simulink library "visionanalysis"  (R2017b)
settings: Solver=ode45  StartTime=0.0  StopTime=10.0  RelTol=1e-3
undefined symbols (not defined in the file or in its folder): dtInfo, fspecial
libraries: visionstatistics x1
settings Model: FPTRunName=Active  ExtModeAutoUpdateStatusClock=off  Creator=The MathWorks, Inc.  LastModifiedBy=The MathWorks, Inc.
settings DataIOCC: LimitDataPoints=on  SaveFormat=Array  SignalLoggingSaveFormat=ModelDataLogs
settings OptimizationCC: BlockReduction=off  BooleanDataType=off  ExpressionDepthLimit=2147483647  EfficientMapNaN2IntZero=off  LifeSpan=inf
settings DebuggingCC: SaveWithParameterizedLinksMsg=none  UnderspecifiedInitializationDetection=Classic  MergeDetectMultiDrivingBlocksExec=none  SignalResolutionControl=TryResolveAllWithWarning  FcnCallInpInsideContextMsg=warning  AllowSymbolicDim=off  StateNameClashWarn=warning  StrictBusMsg=Warning  SFUnexpectedBacktrackingDiag=warning  SFNoUnconditionalDefaultTransitionDiag=warning  SFExecutionAtInitializationDiag=none
settings HardwareCC: ProdBitPerPointer=32  ProdBitPerSizeT=32  ProdBitPerPtrDiffT=32  ProdLargestAtomicFloat=None  ProdIntDivRoundTo=Undefined  ProdEndianess=Unspecified  ProdWordSize=32  ProdHWDeviceType=32-bit Generic  TargetUnknown=on
settings ModelReferenceCC: PropagateSignalLabelsOutOfModel=off
settings CodeAppCC: StateflowObjectComments=on
settings GRTTargetCC: TargetLangStandard=C89/C90 (ANSI)  GeneratePreprocessorConditionals=Disable all  CombineOutputUpdateFcns=off  GRTInterface=on
settings ConfigComp: CovMetricSettings=dw  CovHtmlReporting=on  CovSaveCumulativeToWorkspaceVar=on  CovSaveSingleToWorkspaceVar=on  CovShowResultsExplorer=off  CovExternalEMLEnable=off  CovSFcnEnable=off

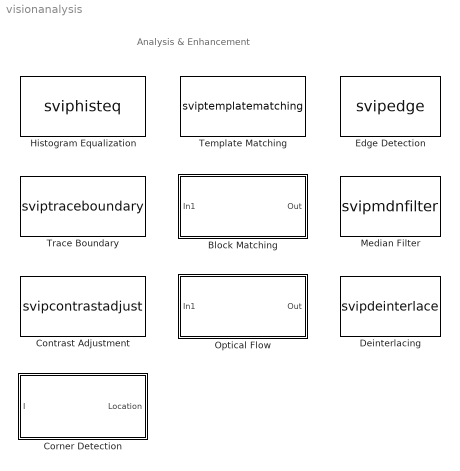
== system visionanalysis ==
  note: Analysis & Enhancement
  Block Matching : Subsystem  DialogController=vipDDGCreate  mask(Block Matching){which2img=Current frame and N-th frame back, N=1, searchMethod=Exhaustive, blockSize=[17 17], overlapping=[0 0], maxDisplacement=[7 7], matchCriteria=Mean square error (MSE), outVelForm=Magnitude-squared, outputMode=Binary point scaling, outputWordLength=8, outputFracLength=0, accumMode=Binary point scaling, accumWordLength=32, accumFracLength=0, prodOutputMode=Binary point scaling, prodOutputWordLength=32, prodOutputFracLength=0, roundingMode=Floor, overflowMode=on, LockScale=off}
      mask prompts: which2img "vision:masks:EstimateMotionBetween"; N "vision:masks:N"; searchMethod "vision:masks:SearchMethod"; blockSize "vision:masks:BlockSizeheightWidth"; overlapping "vision:masks:OverlapSizerC"; maxDisplacement "vision:masks:MaximumDisplacementrC"; matchCriteria "vision:masks:BlockMatchingCriteria"; outVelForm "vision:masks:VelocityOutput"; outputMode "vision:masks:FixedpointOutputAttributes"; outputWordLength "vision:masks:OutputWordLength"; outputFracLength "vision:masks:OutputFractionalLength"; accumMode "vision:masks:FixedpointAccumulatorAttributes"; accumWordLength "vision:masks:AccumulatorWordLength"; accumFracLength "vision:masks:AccumulatorFractionLength"; prodOutputMode "vision:masks:FixedpointProductOutputAttribute"; prodOutputWordLength "vision:masks:ProductOutputWordLength"; prodOutputFracLength "vision:masks:ProductOutputFractionLength"; roundingMode "vision:masks:RoundIntegerCalculationsTowards"; overflowMode "vision:masks:SaturateOnIntegerOverflow"; LockScale "vision:masks:LockScaling1"
      mask help: vision:masks:BlockMatchingDescription
      mask init:
      | [disp_str,si,so]=vipblkblockmatch('icon',which2img);
      | vipblkblockmatch('init');
      mask Help: eval('visionblockhelp');
      mask TypeOptions which2img: vision:masks:TwoImages | vision:masks:CurrentFrameAndNthFrameBack
      mask TypeOptions searchMethod: vision:masks:Exhaustive | vision:masks:Threestep
      mask TypeOptions matchCriteria: vision:masks:MeanSquareErrorMSE | vision:masks:MeanAbsoluteDifferenceMAD
      mask TypeOptions outVelForm: vision:masks:HorizontalAndVerticalComponentsI | vision:masks:Magnitudesquared
      mask TypeOptions outputMode: Binary point scaling | Slope and bias scaling
      mask TypeOptions accumMode: Binary point scaling | Slope and bias scaling
      mask TypeOptions prodOutputMode: Same as input | Binary point scaling | Slope and bias scaling
      mask TypeOptions roundingMode: dspshared:FixptDialog:Ceiling_CB | dspshared:FixptDialog:Convergent_CB | dspshared:FixptDialog:Floor_CB | dspshared:FixptDialog:Nearest_CB | dspshared:FixptDialog:Round_CB | dspshared:FixptDialog:Simplest_CB | dspshared:FixptDialog:Zero_CB
      mask Display:
      | disp(disp_str);
      | port_label('input',si(1).port,si(1).txt);
      | port_label('input',si(2).port,si(2).txt);
      | 
      | port_label('output',1,so(1).txt);
  Contrast Adjustment : S-Function  DialogController=vipDDGCreate  FunctionName=svipcontrastadjust  Parameters=methodInputRange, rangeIn, fracSaturate, isBinNum, binNum, methodOutputRange, rangeOut, prod1Mode, prod1WordLength, prod1FracLength, prod2Mode, prod2WordLength, prod2FracLength, dtInfo.roundingMode, dtInfo.overflowMode  SFunctionDeploymentMode=off  EnableBusSupport=off  mask(Contrast Adjustment){methodInputRange=Full input data range [min max], rangeIn=[0 255], fracSaturate=[1 1], isBinNum=on, binNum=256, methodOutputRange=Full data type range, rangeOut=[0 255], prod1Mode=Binary point scaling, prod1WordLength=32, prod1FracLength=16, prod2Mode=Binary point scaling, prod2WordLength=32, prod2FracLength=16, roundingMode=Floor, overflowMode=off, LockScale=off}
      mask prompts: methodInputRange "vision:masks:AdjustPixelValuesFrom"; rangeIn "vision:masks:RangelowHigh"; fracSaturate "vision:masks:PercentageOfPixelsToSaturatelowH"; isBinNum "vision:masks:SpecifyNumberOfHistogramBinsused"; binNum "vision:masks:NumberOfHistogramBins"; methodOutputRange "vision:masks:AdjustPixelValuesTo"; rangeOut "vision:masks:RangelowHigh"; prod1Mode "vision:masks:Product1Attributes"; prod1WordLength "vision:masks:Product1WordLength"; prod1FracLength "vision:masks:Product1FractionLength"; prod2Mode "vision:masks:Product2Attributes"; prod2WordLength "vision:masks:Product2WordLength"; prod2FracLength "vision:masks:Product2FractionLength"; roundingMode "vision:masks:RoundIntegerCalculationsToward"; overflowMode "vision:masks:SaturateOnIntegerOverflow"; LockScale "vision:masks:LockScaling1"
      mask help: vision:masks:ContrastAdjustmentDescription
      mask init:
      | dtInfo = dspGetFixptDataTypeInfo(gcbh,1);
      | fracSaturate = single(fracSaturate) ./ single(100);
      mask Help: eval('visionblockhelp');
      mask TypeOptions methodInputRange: vision:masks:FullInputDataRangeminMax | vision:masks:UserdefinedRange | vision:masks:RangeDeterminedBySaturating
      mask TypeOptions methodOutputRange: vision:masks:FullDataTypeRange | vision:masks:UserdefinedRange
      mask TypeOptions prod1Mode: Binary point scaling | Slope and bias scaling
      mask TypeOptions prod2Mode: Binary point scaling | Slope and bias scaling
      mask TypeOptions roundingMode: dspshared:FixptDialog:Ceiling_CB | dspshared:FixptDialog:Convergent_CB | dspshared:FixptDialog:Floor_CB | dspshared:FixptDialog:Nearest_CB | dspshared:FixptDialog:Round_CB | dspshared:FixptDialog:Simplest_CB | dspshared:FixptDialog:Zero_CB
      mask Display:
      | disp('Contrast\nAdjustment');
      | port_label('input',1,'I');
  Corner Detection : Subsystem  DialogController=vipDDGCreate  mask(Corner Detection){method=Harris corner detection (Harris & Stephens), factor=0.04, filter=fspecial('gaussian', [1 5], 1.5), thrInten=0.1, thrAngle=157.5, output=Obsolete9b, outputInUse=Corner location, maxNum=200, thrMetric=0.0005, neighborSize=[11 11], isOutVarDim=on, outputMode=Same as accumulator, outputWordLength=32, outputFracLength=0, accumMode=Binary point scaling, accumWordLength=32, accumFracLength=0, prodOutputMode=Binary point scaling, prodOutputWordLength=32, prodOutputFracLength=0, memoryMode=Binary point scaling, memoryWordLength=32, memoryFracLength=0, firstCoeffMode=Specify word length, firstCoeffWordLength=16, firstCoeffFracLength=16, roundingMode=Floor, overflowMode=off, LockScale=off}
      mask prompts: method "vision:masks:Method"; factor "vision:masks:SensitivityFactor"; filter "vision:masks:CoefficientsSeparableSmoothing"; thrInten "vision:masks:IntensityComparisonThreshold"; thrAngle "vision:masks:MaximumAngleToBeConsidered"; output "dspshared:FixptDialog:Output_MP"; outputInUse "dspshared:FixptDialog:Output_MP"; maxNum "vision:masks:MaximumNumberOfCorners"; thrMetric "vision:masks:MinimumMetricValueThatIndicates"; neighborSize "vision:masks:NeighborhoodSizesuppressRegion"; isOutVarDim "vision:masks:OutputVariableSizeSignal"; outputMode "vision:masks:OutputAttributes"; outputWordLength "vision:masks:OutputWordLength"; outputFracLength "vision:masks:OutputFractionalLength"; accumMode "vision:masks:AccumulatorAttributes"; accumWordLength "vision:masks:AccumulatorWordLength"; accumFracLength "vision:masks:AccumulatorFractionLength"; prodOutputMode "vision:masks:ProductOutputAttributes"; prodOutputWordLength "vision:masks:ProductOutputWordLength"; prodOutputFracLength "vision:masks:ProductOutputFractionLength"; memoryMode "vision:masks:MemoryAttributes"; memoryWordLength "vision:masks:MemoryWordLength"; memoryFracLength "vision:masks:MemoryFractionLength"; firstCoeffMode "vision:masks:FirstCoefficientAttributes"; firstCoeffWordLength "vision:masks:FirstCoefficientWordLength"; firstCoeffFracLength "vision:masks:FirstCoefficientFractionLength"; roundingMode "vision:masks:RoundIntegerCalculationsToward"; overflowMode "vision:masks:SaturateOnIntegerOverflow"; LockScale "vision:masks:LockScaling1"
      mask help: vision:masks:CornerDetectionDescription
      mask init:
      | blkh = gcbh;
      | dtInfo = dspGetFixptDataTypeInfo(blkh, 63); %63
      | outport = vipblkcornerdetection(blkh, output, outputInUse, isOutVarDim);
      mask Help: eval('visionblockhelp');
      mask TypeOptions method: vision:masks:HarrisCornerDetectionHarrisSteph | vision:masks:MinimumEigenvalueShiTomasi | vision:masks:LocalIntensityComparisonRosenDr
      mask TypeOptions thrAngle: 22.5 | 45.0 | 67.5 | 90.0 | 112.5 | 135.0 | 157.5
      mask TypeOptions output: vision:masks:CornerLocation | vision:masks:CornerLocationAndMetricMatrix | vision:masks:MetricMatrix | vision:masks:Obsolete9b
      mask TypeOptions outputInUse: vision:masks:CornerLocation | vision:masks:CornerLocationAndMetricMatrix | vision:masks:MetricMatrix
      mask TypeOptions outputMode: Same as accumulator | Same as input | Binary point scaling | Slope and bias scaling
      mask TypeOptions accumMode: Same as input | Binary point scaling | Slope and bias scaling
      mask TypeOptions prodOutputMode: Same as input | Binary point scaling | Slope and bias scaling
      mask TypeOptions memoryMode: Same as input | Binary point scaling | Slope and bias scaling
      mask TypeOptions firstCoeffMode: Same word length as input | Specify word length | Binary point scaling | Slope and bias scaling
      mask TypeOptions roundingMode: dspshared:FixptDialog:Ceiling_CB | dspshared:FixptDialog:Convergent_CB | dspshared:FixptDialog:Floor_CB | dspshared:FixptDialog:Nearest_CB | dspshared:FixptDialog:Round_CB | dspshared:FixptDialog:Simplest_CB | dspshared:FixptDialog:Zero_CB
      mask Display:
      | disp('Corner\nDetection');
      | port_label('input',1,'I');
      | port_label('output', outport(1).port, outport(1).txt);
      | port_label('output', outport(2).port, outport(2).txt);
      | port_label('output', outport(3).port, outport(3).txt);
  Deinterlacing : S-Function  DialogController=vipDDGCreate  FunctionName=svipdeinterlace  Parameters=method,isInputTransposed,dtInfo.accumMode,dtInfo.accumWordLength,dtInfo.accumFracLength,dtInfo.outputMode,dtInfo.outputWordLength,dtInfo.outputFracLength,dtInfo.roundingMode,dtInfo.overflowMode  SFunctionDeploymentMode=off  EnableBusSupport=off  mask(Deinterlacing){method=Line repetition, isInputTransposed=off, outputMode=Same as input, outputWordLength=8, outputFracLength=0, accumMode=Binary point scaling, accumWordLength=12, accumFracLength=3, prodOutputMode=Binary point scaling, prodOutputWordLength=12, prodOutputFracLength=3, roundingMode=Floor, overflowMode=on, LockScale=off}
      mask prompts: method "vision:masks:Method"; isInputTransposed "vision:masks:InputImageIsTransposed"; outputMode "vision:masks:FixedpointOutputAttributes"; outputWordLength "vision:masks:OutputWordLength"; outputFracLength "vision:masks:OutputFractionalLength"; accumMode "vision:masks:FixedpointAccumulatorAttributes"; accumWordLength "vision:masks:AccumulatorWordLength"; accumFracLength "vision:masks:AccumulatorFractionLength"; prodOutputMode "vision:masks:FixedpointProductOutputAttribute"; prodOutputWordLength "vision:masks:ProductOutputWordLength"; prodOutputFracLength "vision:masks:ProductOutputFractionLength"; roundingMode "vision:masks:RoundIntegerCalculationsTowards"; overflowMode "vision:masks:SaturateOnIntegerOverflow"; LockScale "vision:masks:LockScaling1"
      mask help: vision:masks:DeinterlacingDescription
      mask init:
      | dtInfo = dspGetFixptDataTypeInfo(gcbh,7);
      mask Help: eval('visionblockhelp');
      mask TypeOptions method: vision:masks:LineRepetition | vision:masks:LinearInterpolation | vision:masks:VerticalTemporalMedianFiltering
      mask TypeOptions outputMode: Same as input | Binary point scaling | Slope and bias scaling
      mask TypeOptions accumMode: Same as input | Binary point scaling | Slope and bias scaling
      mask TypeOptions prodOutputMode: Same as input | Binary point scaling | Slope and bias scaling
      mask TypeOptions roundingMode: dspshared:FixptDialog:Ceiling_CB | dspshared:FixptDialog:Convergent_CB | dspshared:FixptDialog:Floor_CB | dspshared:FixptDialog:Nearest_CB | dspshared:FixptDialog:Round_CB | dspshared:FixptDialog:Simplest_CB | dspshared:FixptDialog:Zero_CB
      mask Display: disp('Deinterlacing')
  Edge Detection : S-Function  DialogController=vipDDGCreate  FunctionName=svipedge  Parameters=method, outputType, userDefinedThreshold, thresholdSource, threshold, thresholdTuning, edgeThinning,threshold_canny,autoPercent,sigma,dtInfo. prodOutputMode,dtInfo.prodOutputWordLength,dtInfo.prodOutputFracLength,dtInfo.accumMode,dtInfo.accumWordLength,dtInfo.accumFracLength,dtInfo.outputMode,dtInfo.outputWordLength,dtInfo.outputFracLength,dtInfo.roundingMode,dtInfo.overflowMode  SFunctionDeploymentMode=off  EnableBusSupport=off  mask(Edge Detection){method=Sobel, outputType=Binary image, userDefinedThreshold=off, thresholdSource=Input port, threshold=20, thresholdTuning=4, edgeThinning=off, threshold_canny=[0.25 0.60], autoPercent=70, sigma=1, outputMode=Same as first input, outputWordLength=16, outputFracLength=4, accumMode=Same as product output, accumWordLength=32, accumFracLength=8, prodOutputMode=Binary point scaling, prodOutputWordLength=32, prodOutputFracLength=8, roundingMode=Floor, overflowMode=off, LockScale=off}
      mask prompts: method "vision:masks:Method"; outputType "vision:masks:OutputType"; userDefinedThreshold "vision:masks:UserdefinedThreshold"; thresholdSource "vision:masks:ThresholdSource"; threshold "vision:masks:Threshold"; thresholdTuning "vision:masks:ThresholdScaleFactor_1"; edgeThinning "vision:masks:EdgeThinning"; threshold_canny "vision:masks:ThresholdLowHigh"; autoPercent "vision:masks:PercentOfPixelsNotEdges"; sigma "vision:masks:Sigma"; outputMode "vision:masks:FixedpointOutputAttributes"; outputWordLength "vision:masks:OutputWordLength"; outputFracLength "vision:masks:OutputFractionLength"; accumMode "vision:masks:FixedpointAccumulatorAttributes"; accumWordLength "vision:masks:AccumulatorWordLength"; accumFracLength "vision:masks:AccumulatorFractionLength"; prodOutputMode "vision:masks:FixedpointProductOutputAttribute"; prodOutputWordLength "vision:masks:ProductOutputWordLength"; prodOutputFracLength "vision:masks:ProductOutputFractionLength"; roundingMode "vision:masks:RoundIntegerCalculationsTowards"; overflowMode "vision:masks:SaturateOnIntegerOverflow"; LockScale "vision:masks:LockScaling1"
      mask help: vision:masks:EdgeDetectionDescription
      mask init:
      | [si,so,blkname,dtInfo]= vipblkedge;
      mask Help: eval('visionblockhelp');
      mask TypeOptions method: vision:masks:Sobel | vision:masks:Prewitt | vision:masks:Roberts | vision:masks:Canny
      mask TypeOptions outputType: vision:masks:BinaryImage | vision:masks:GradientComponents | vision:masks:BinaryImageAndGradientComponents
      mask TypeOptions thresholdSource: vision:masks:SpecifyViaDialog | vision:masks:InputPort
      mask TypeOptions outputMode: Same as accumulator | Same as product output | Same as first input | Binary point scaling | Slope and bias scaling
      mask TypeOptions accumMode: Same as product output | Same as first input | Binary point scaling | Slope and bias scaling
      mask TypeOptions prodOutputMode: Same as first input | Binary point scaling | Slope and bias scaling
      mask TypeOptions roundingMode: dspshared:FixptDialog:Ceiling_CB | dspshared:FixptDialog:Convergent_CB | dspshared:FixptDialog:Floor_CB | dspshared:FixptDialog:Nearest_CB | dspshared:FixptDialog:Round_CB | dspshared:FixptDialog:Simplest_CB | dspshared:FixptDialog:Zero_CB
      mask Display:
      | disp(blkname)
      | 
      | port_label('input', si(1).port, si(1).txt);
      | port_label('input', si(2).port, si(2).txt);
      | 
      | port_label('output',so(1).port, so(1).txt);
      | port_label('output',so(2).port, so(2).txt);
      | port_label('output',so(3).port, so(3).txt);
  Histogram Equalization : S-Function  FunctionName=sviphisteq  Parameters=specify, numbins, src, hist  SFunctionDeploymentMode=off  EnableBusSupport=off  mask(Histogram Equalization){specify=Uniform, numbins=64, src=Specify via dialog, hist=ones(1,64)}
      mask prompts: specify "vision:masks:TargetHistogram"; numbins "vision:masks:NumberOfBins"; src "vision:masks:HistogramSource"; hist "vision:masks:Histogram"
      mask help: vision:masks:HistogramEqualizationDescription
      mask init:
      | ports(1).num = 1;
      | ports(1).txt = 'I';
      | if (specify == 2 && src == 2)
      | 	ports(2).num = 2;
      | 	ports(2).txt = 'Hist';
      | else
      | 	ports(2).num = 1;
      | 	ports(2).txt = 'I';
      | end
      mask Help: eval('visionblockhelp');
      mask TypeOptions specify: vision:masks:Uniform | vision:masks:Userdefined
      mask Callback specify:
      | if (strcmp(get_param(gcbh,'specify'),'Uniform'))
      | 	set_param(gcbh,'MaskVisibilities',{'on','on','off','off'});
      | else
      | 	if (strcmp(get_param(gcbh,'src'),'Input port'))
      | 		set_param(gcbh,'MaskVisibilities',{'on','off','on','off'});
      | 	else
      | 		set_param(gcbh,'MaskVisibilities',{'on','off','on','on'});
      | 	end
      | end
      mask TypeOptions src: vision:masks:SpecifyViaDialog | vision:masks:InputPort
      mask Callback src:
      | if (strcmp(get_param(gcbh,'specify'),'User-defined'))
      | 	if (strcmp(get_param(gcbh,'src'),'Input port'))
      | 		set_param(gcbh,'MaskVisibilities',{'on','off','on','off'});
      | 	else
      | 		set_param(gcbh,'MaskVisibilities',{'on','off','on','on'});
      | 	end
      | end
      mask Display:
      | disp('Histogram\nEqualization');
      | 
      | port_label('input',ports(1).num,ports(1).txt);
      | port_label('input',ports(2).num,ports(2).txt);
  Median Filter : S-Function  DialogController=vipDDGCreate  FunctionName=svipmdnfilter  Parameters=nghbood,outSize,padType,padSrc,padVal,dtInfo.accumMode,dtInfo.accumWordLength,dtInfo.accumFracLength,dtInfo.outputMode,dtInfo.outputWordLength,dtInfo.outputFracLength,dtInfo.roundingMode,dtInfo.overflowMode  SFunctionDeploymentMode=off  EnableBusSupport=on  mask(Median Filter){nghbood=[3 3], outSize=Same as input port I, padType=Constant, padSrc=Specify via dialog, padVal=0, outputMode=Same as input, outputWordLength=16, outputFracLength=15, accumMode=Same as input, accumWordLength=32, accumFracLength=30, prodOutputMode=Same as input, prodOutputWordLength=32, prodOutputFracLength=30, roundingMode=Floor, overflowMode=off, LockScale=off}
      mask prompts: nghbood "vision:masks:NeighborhoodSize"; outSize "vision:masks:OutputSize"; padType "vision:masks:PaddingOptions"; padSrc "vision:masks:PadValueSource"; padVal "vision:masks:PadValue"; outputMode "vision:masks:FixedpointOutputAttributes"; outputWordLength "vision:masks:OutputWordLength"; outputFracLength "vision:masks:OutputFractionalLength"; accumMode "vision:masks:FixedpointAccumulatorAttributes"; accumWordLength "vision:masks:AccumulatorWordLength"; accumFracLength "vision:masks:AccumulatorFractionLength"; prodOutputMode "vision:masks:FixedpointProductOutputAttribute"; prodOutputWordLength "vision:masks:ProductOutputWordLength"; prodOutputFracLength "vision:masks:ProductOutputFractionLength"; roundingMode "vision:masks:RoundIntegerCalculationsTowards"; overflowMode "vision:masks:SaturateOnIntegerOverflow"; LockScale "vision:masks:LockScaling1"
      mask help: vision:masks:MedianFilterDescription
      mask init:
      | [ports,dtInfo] = vipblkmdnfilter;
      mask Help: eval('visionblockhelp');
      mask TypeOptions outSize: vision:masks:SameAsInputPortI | vision:masks:Valid
      mask TypeOptions padType: vision:masks:Constant | vision:masks:Replicate | vision:masks:Symmetric | vision:masks:Circular
      mask TypeOptions padSrc: vision:masks:SpecifyViaDialog | vision:masks:InputPort
      mask TypeOptions outputMode: Same as input | Binary point scaling | Slope and bias scaling
      mask TypeOptions accumMode: Same as input | Binary point scaling | Slope and bias scaling
      mask TypeOptions prodOutputMode: Same as input | Binary point scaling | Slope and bias scaling
      mask TypeOptions roundingMode: dspshared:FixptDialog:Ceiling_CB | dspshared:FixptDialog:Convergent_CB | dspshared:FixptDialog:Floor_CB | dspshared:FixptDialog:Nearest_CB | dspshared:FixptDialog:Round_CB | dspshared:FixptDialog:Simplest_CB | dspshared:FixptDialog:Zero_CB
      mask Display:
      | disp('Median\n Filter');
      | port_label('input',ports.port1, ports.txt1);
      | port_label('input',ports.port2, ports.txt2);
      | port_label('output',ports.port3, ports.txt3);
  Optical Flow : Subsystem  DialogController=vipDDGCreate  mask(Optical Flow){method=Horn-Schunck, gradMethod=Difference filter [-1 1], which2img=Current frame and N-th frame back, N=1, outVelForm=Magnitude-squared, lambda=1, stop_criteria=When maximum number of iterations is reached, maxAllowAbsDiff=eps, maxIter=10, numInports=3, sigmaS=1.5, sigmaW=1, eigTh=0.0039, discardNormalFlow=off, outputCurrentImage=off, firstCoeffMode=Same word length as first input, firstCoeffWordLength=16, firstCoeffFracLength=12, prodOutputMode=Binary point scaling, prodOutputWordLength=32, prodOutputFracLength=20, accumMode=Same as product output, accumWordLength=32, accumFracLength=20, memoryMode=Same as accumulator, memoryWordLength=32, memoryFracLength=20, outputMode=Binary point scaling, outputWordLength=32, outputFracLength=20, roundingMode=Nearest, overflowMode=on, LockScale=off}
      mask prompts: method "vision:masks:Method"; gradMethod "vision:masks:GradientMethod"; which2img "vision:masks:ComputeOpticalFlowBetween"; N "vision:masks:N"; outVelForm "vision:masks:VelocityOutput"; lambda "vision:masks:SmoothnessFactor"; stop_criteria "vision:masks:StopIterativeSolution"; maxAllowAbsDiff "vision:masks:VelocityDifferenceThreshold"; maxIter "vision:masks:MaximumNumberOfIterations"; numInports "vision:masks:NumberOfInputFramesToBuffer"; sigmaS "vision:masks:SDForImageSmoothing"; sigmaW "vision:masks:SDForGradientSmoothing"; eigTh "vision:masks:ThresholdForNoiseReduction"; discardNormalFlow "vision:masks:DiscardNormalFlowEstimates"; outputCurrentImage "vision:masks:OutputImageCorrespondingToMotion"; firstCoeffMode "vision:masks:EigenThresholdAttributes"; firstCoeffWordLength "vision:masks:EigenThresholdWordLength"; firstCoeffFracLength "vision:masks:EigenThresholdFractionLength"; prodOutputMode "vision:masks:ProductOutputAttributes"; prodOutputWordLength "vision:masks:ProductOutputWordLength"; prodOutputFracLength "vision:masks:ProductOutputFractionLength"; accumMode "vision:masks:AccumulatorAttributes"; accumWordLength "vision:masks:AccumulatorWordLength"; accumFracLength "vision:masks:AccumulatorFractionLength"; memoryMode "vision:masks:GradientAttributes"; memoryWordLength "vision:masks:GradientWordLength"; memoryFracLength "vision:masks:GradientFractionLength"; outputMode "vision:masks:FixedpointOutputAttributes"; outputWordLength "vision:masks:OutputWordLength"; outputFracLength "vision:masks:OutputFractionalLength"; roundingMode "vision:masks:RoundIntegerCalculationsToward"; overflowMode "vision:masks:SaturateOnIntegerOverflow"; LockScale "vision:masks:LockScaling1"
      mask help: vision:masks:OpticalFlowDescription
      mask init:
      | [disp_str,si,so]=vipblkopticalflow(which2img,double(numInports));
      mask Help: eval('visionblockhelp');
      mask TypeOptions method: vision:masks:HornSchunck | vision:masks:LucasKanade
      mask TypeOptions gradMethod: vision:masks:DerivativeOfGaussian | vision:masks:DifferenceFilter
      mask TypeOptions which2img: vision:masks:TwoImages | vision:masks:CurrentFrameAndNthFrameBack
      mask TypeOptions outVelForm: vision:masks:HorizontalAndVerticalComponentsI | vision:masks:Magnitudesquared
      mask TypeOptions stop_criteria: vision:masks:WhenVelocityDifferenceFallsBelow | vision:masks:WhenMaximumNumberOfIterations | vision:masks:WhicheverComesFirst
      mask TypeOptions firstCoeffMode: dspshared:FixptDialog:SameWordLengthAsFirstInput | dspshared:FixptDialog:SpecifyWordLength | dspshared:FixptDialog:BinaryPointScaling | dspshared:FixptDialog:SlopeAndBiasScaling
      mask TypeOptions prodOutputMode: dspshared:FixptDialog:BinaryPointScaling | dspshared:FixptDialog:SlopeAndBiasScaling
      mask TypeOptions accumMode: dspshared:FixptDialog:SameAsProductOutput | dspshared:FixptDialog:BinaryPointScaling | dspshared:FixptDialog:SlopeAndBiasScaling
      mask TypeOptions memoryMode: dspshared:FixptDialog:SameAsAccumulator | dspshared:FixptDialog:SameAsProductOutput | dspshared:FixptDialog:BinaryPointScaling | dspshared:FixptDialog:SlopeAndBiasScaling
      mask TypeOptions outputMode: dspshared:FixptDialog:BinaryPointScaling | dspshared:FixptDialog:SlopeAndBiasScaling
      mask TypeOptions roundingMode: dspshared:FixptDialog:Ceiling_CB | dspshared:FixptDialog:Convergent_CB | dspshared:FixptDialog:Floor_CB | dspshared:FixptDialog:Nearest_CB | dspshared:FixptDialog:Round_CB | dspshared:FixptDialog:Simplest_CB | dspshared:FixptDialog:Zero_CB
      mask Display:
      | disp(disp_str);
      | port_label('input',si(1).port,si(1).txt);
      | port_label('input',si(2).port,si(2).txt);
      | 
      | port_label('output',so(1).port,so(1).txt);
      | port_label('output',so(2).port,so(2).txt);
  Template Matching : S-Function  DialogController=vipDDGCreate  FunctionName=sviptemplatematching  Parameters=metric,output,method,nMetric,nSize,roi,roiValid,dtInfo.prodOutputMode,dtInfo.prodOutputWordLength,dtInfo.prodOutputFracLength,dtInfo.accumMode,dtInfo.accumWordLength,dtInfo.accumFracLength,dtInfo.outputMode,dtInfo.outputWordLength,dtInfo.outputFracLength,dtInfo.roundingMode,dtInfo.overflowMode  SFunctionDeploymentMode=off  EnableBusSupport=off  mask(Template Matching){metric=Sum of absolute differences, output=Best match location, method=Exhaustive, nMetric=off, nSize=3, roi=off, roiValid=off, outputMode=Same as first input, outputWordLength=32, outputFracLength=0, accumMode=Binary point scaling, accumWordLength=32, accumFracLength=0, prodOutputMode=Binary point scaling, prodOutputWordLength=32, prodOutputFracLength=0, roundingMode=Floor, overflowMode=off, LockScale=off}
      mask prompts: metric "vision:masks:MatchMetric1"; output "dspshared:FixptDialog:Output_MP"; method "vision:masks:SearchMethod"; nMetric "vision:masks:OutputNxNMatrixOfMetricValues"; nSize "vision:masks:SizeNOfSquareMatrix"; roi "vision:masks:EnableROIProcessing"; roiValid "vision:masks:OutputFlagIndicatingIfROIIsValid"; outputMode "vision:masks:FixedpointOutputAttributes"; outputWordLength "vision:masks:OutputWordLength"; outputFracLength "vision:masks:OutputFractionalLength"; accumMode "vision:masks:FixedpointAccumulatorAttributes"; accumWordLength "vision:masks:AccumulatorWordLength"; accumFracLength "vision:masks:AccumulatorFractionLength"; prodOutputMode "vision:masks:FixedpointProductAttributes"; prodOutputWordLength "vision:masks:ProductWordLength"; prodOutputFracLength "vision:masks:ProductFractionLength"; roundingMode "vision:masks:RoundIntegerCalculationsTowards"; overflowMode "vision:masks:SaturateOnIntegerOverflow"; LockScale "vision:masks:LockScaling1"
      mask help: vision:masks:TemplateMatchingDescription
      mask init:
      | [ports blkname]    = vipblktemplatematching('icon');
      | dtInfo   = vipblktemplatematching('init');
      mask Help: eval('visionblockhelp');
      mask TypeOptions metric: vision:masks:SumOfAbsoluteDifferences | vision:masks:SumOfSquaredDifferences | vision:masks:MaximumAbsoluteDifference
      mask Callback metric: vipblktemplatematching
      mask TypeOptions output: vision:masks:MetricMatrix | vision:masks:BestMatchLocation
      mask Callback output: vipblktemplatematching
      mask TypeOptions method: vision:masks:Exhaustive | vision:masks:Threestep
      mask Callback method: vipblktemplatematching
      mask Callback nMetric: vipblktemplatematching
      mask Callback nSize: vipblktemplatematching
      mask Callback roi: vipblktemplatematching
      mask Callback roiValid: vipblktemplatematching
      mask TypeOptions outputMode: Same as first input | Binary point scaling | Slope and bias scaling
      mask TypeOptions accumMode: Same as first input | Binary point scaling | Slope and bias scaling
      mask TypeOptions prodOutputMode: Same as first input | Binary point scaling | Slope and bias scaling
      mask TypeOptions roundingMode: dspshared:FixptDialog:Ceiling_CB | dspshared:FixptDialog:Convergent_CB | dspshared:FixptDialog:Floor_CB | dspshared:FixptDialog:Nearest_CB | dspshared:FixptDialog:Round_CB | dspshared:FixptDialog:Simplest_CB | dspshared:FixptDialog:Zero_CB
      mask Display:
      | disp(blkname)
      | port_label('input',ports.iport1, ports.itxt1);
      | port_label('input',ports.iport2, ports.itxt2);
      | port_label('input',ports.iport3, ports.itxt3);
      | port_label('output',ports.oport1, ports.otxt1);
      | port_label('output',ports.oport2, ports.otxt2);
      | port_label('output',ports.oport3, ports.otxt3);
      | port_label('output',ports.oport4, ports.otxt4);
  Trace Boundary : S-Function  FunctionName=sviptraceboundary  Parameters=conn,searchDir4,searchDir8,traceDir,maxNumPix,outputNum,fillChoices,fillVal  SFunctionDeploymentMode=off  EnableBusSupport=off  mask(Trace Boundary){conn=8, searchDir4=North, searchDir8=North, traceDir=Clockwise, maxNumPix=500, outputNum=off, fillChoices=None, fillVal=[0 0]}
      mask prompts: conn "vision:masks:Connectivity"; searchDir4 "vision:masks:InitialSearchDirection"; searchDir8 "vision:masks:InitialSearchDirection"; traceDir "vision:masks:TraceDirection"; maxNumPix "vision:masks:MaximumNumberOfBoundaryPixels"; outputNum "vision:masks:OutputNumberOfBoundaryPixels"; fillChoices "vision:masks:ActionToTakeForEmptyOutputPoints"; fillVal "vision:masks:FillValues"
      mask help: vision:masks:TraceBoundaryDescription
      mask init:
      | so = vipblkboundarytracing('icon2');
      mask Help: eval('visionblockhelp');
      mask TypeOptions conn: 4 | 8
      mask Callback conn: vipblkboundarytracing('dynamic2');
      mask TypeOptions searchDir4: vision:masks:North | vision:masks:East | vision:masks:South | vision:masks:West
      mask TypeOptions searchDir8: vision:masks:North | vision:masks:Northeast | vision:masks:East | vision:masks:Southeast | vision:masks:South | vision:masks:Southwest | vision:masks:West | vision:masks:Northwest
      mask TypeOptions traceDir: vision:masks:Clockwise | vision:masks:Counterclockwise
      mask TypeOptions fillChoices: vision:masks:None | vision:masks:FillWithLastPointFound | vision:masks:FillWithUserdefinedValues
      mask Display:
      | disp(['Trace\nBoundary']);
      | port_label('input',1,'BW');
      | port_label('input',2,'Start Pt');
      | port_label('output',so(1).port, so(1).txt);
      | port_label('output',so(2).port, so(2).txt);

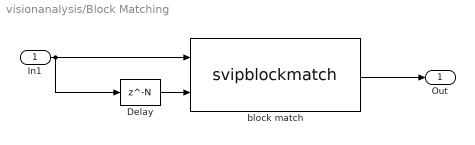
== system visionanalysis/Block Matching ==
  In1 : Inport
  Delay : Delay  DelayLength=N
  block match : S-Function  DialogController=vipDDGCreate  FunctionName=svipblockmatch  Parameters=searchMethod,blockSize,overlapping,maxDisplacement,matchCriteria,outVelForm,dtInfo.prodOutputMode,dtInfo.prodOutputWordLength,dtInfo.prodOutputFracLength,dtInfo.accumMode,dtInfo.accumWordLength,dtInfo.accumFracLength,dtInfo.outputMode,dtInfo.outputWordLength,dtInfo.outputFracLength,dtInfo.roundingMode,dtInfo.overflowMode  SFunctionDeploymentMode=off  EnableBusSupport=off  mask(block match){which2img=Two images, N=1, searchMethod=Exhaustive, blockSize=blockSize, overlapping=overlapping, maxDisplacement=maxDisplacement, matchCriteria=Mean square error (MSE), outVelForm=Magnitude-squared, outputMode=Binary point scaling, outputWordLength=outputWordLength, outputFracLength=outputFracLength, accumMode=Binary point scaling, accumWordLength=accumWordLength, accumFracLength=accumFracLength, prodOutputMode=Binary point scaling, prodOutputWordLength=prodOutputWordLength, prodOutputFracLength=prodOutputFracLength, roundingMode=Floor, overflowMode=on, LockScale=off}
      mask prompts: which2img "Estimate motion between:"; searchMethod "Search method:"; blockSize "Block size [height width]:"; overlapping "Overlap size [r c]:"; maxDisplacement "Maximum displacement [r c]:"; matchCriteria "Block matching criteria:"; outVelForm "Velocity output:"; outputMode "Fixed-point output attributes:"; outputWordLength "Output word length:"; outputFracLength "Output fractional length:"; accumMode "Fixed-point accumulator attributes:"; accumWordLength "Accumulator word length:"; accumFracLength "Accumulator fraction length:"; prodOutputMode "Fixed-point product output attributes:"; prodOutputWordLength "Product output word length:"; prodOutputFracLength "Product output fraction length:"; roundingMode "Round integer calculations towards:"; overflowMode "Saturate on integer overflow"; LockScale "Lock scaling"
      mask help: Estimates motion between two images or two video frames using block matching method.
      mask init:
      | dtInfo = dspGetFixptDataTypeInfo(gcbh,15);
      mask TypeOptions which2img: Two images | Current frame and N-th frame back
      mask TypeOptions searchMethod: Exhaustive | Three-step
      mask TypeOptions matchCriteria: Mean square error (MSE) | Mean absolute difference (MAD)
      mask TypeOptions outVelForm: Horizontal and vertical components in complex form | Magnitude-squared
      mask TypeOptions outputMode: Binary point scaling | Slope and bias scaling
      mask TypeOptions accumMode: Binary point scaling | Slope and bias scaling
      mask TypeOptions prodOutputMode: Same as input | Binary point scaling | Slope and bias scaling
      mask TypeOptions roundingMode: Ceiling | Convergent | Floor | Nearest | Round | Simplest | Zero
  Out : Outport
  wires:
  In1/1 -> block match/1, Delay/1
  block match/1 -> Out/1
  Delay/1 -> block match/2

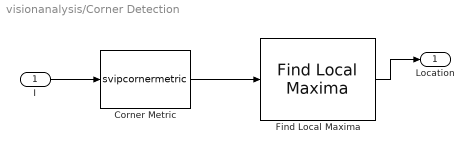
== system visionanalysis/Corner Detection ==
  I : Inport
  Corner Metric : S-Function  DialogController=vipDDGCreate  FunctionName=svipcornermetric  Parameters=method, factor, filter, thrInten, thrAngle, output, outputInUse, maxNum, thrMetric, neighborSize, dtInfo.firstCoeffMode,dtInfo.firstCoeffWordLength,dtInfo.firstCoeffFracLength,dtInfo. prodOutputMode,dtInfo.prodOutputWordLength,dtInfo.prodOutputFracLength,dtInfo.accumMode,dtInfo.accumWordLength,dtInfo.accumFracLength,dtInfo.memoryMode,dtInfo.memoryWordLength,dtInfo.memoryFracLength,dtInfo.outputMode,dtInfo.outputWordLength,dtInfo.outputFracLength,dtInfo.roundingMode,dtInfo.overflowMode  SFunctionDeploymentMode=off  EnableBusSupport=off  mask(Corner Metric){method=Harris corner detection (Harris & Stephens), factor=factor, filter=reshape([filter(:), filter(:)], [2*length(filter), 1]), thrInten=thrInten, thrAngle=157.5, output=Obsolete9b, outputInUse=Corner location, maxNum=maxNum, thrMetric=thrMetric, neighborSize=neighborSize, isOutVarDim=off, outputMode=Same as accumulator, outputWordLength=outputWordLength, outputFracLength=outputFracLength, accumMode=Binary point scaling, accumWordLength=accumWordLength, accumFracLength=accumFracLength, prodOutputMode=Binary point scaling, prodOutputWordLength=prodOutputWordLength, prodOutputFracLength=prodOutputFracLength, memoryMode=Binary point scaling, memoryWordLength=memoryWordLength, memoryFracLength=memoryFracLength, firstCoeffMode=Specify word length, firstCoeffWordLength=firstCoeffWordLength, firstCoeffFracLength=firstCoeffFracLength, roundingMode=Floor, overflowMode=off, LockScale=off}
      mask prompts: factor "Sensitivity factor (0<k<0.25):"; filter "Coefficients for separable smoothing filter:"; thrInten "Intensity comparison threshold:"; thrAngle "Maximum angle to be considered a corner (in degrees):"; outputInUse "Output:"; maxNum "Maximum number of corners:"; thrMetric "Minimum metric value that indicates a corner:"; neighborSize "Neighborhood size (suppress region around detected corners):"; isOutVarDim "Output variable size signal"; outputMode "Output attributes:"; outputWordLength "Output word length:"; outputFracLength "Output fractional length:"; accumMode "Accumulator attributes:"; accumWordLength "Accumulator word length:"; accumFracLength "Accumulator fraction length:"; prodOutputMode "Product output attributes:"; prodOutputWordLength "Product output word length:"; prodOutputFracLength "Product output fraction length:"; memoryMode "Memory attributes:"; memoryWordLength "Memory word length:"; memoryFracLength "Memory fraction length:"; firstCoeffMode "First coefficient attributes:"; firstCoeffWordLength "First coefficient word length:"; firstCoeffFracLength "First coefficient fraction length:"; roundingMode "Round integer calculations toward:"; overflowMode "Saturate on integer overflow"; LockScale "Lock scaling"
      mask help: Calculates the corner metric matrix. This is not a stand alone block: please do not change parameters.
      mask init:
      | blkh = gcbh;
      | dtInfo = dspGetFixptDataTypeInfo(blkh, 63);
      mask Help: eval('visionblockhelp');
      mask TypeOptions method: vision:masks:HarrisCornerDetectionHarrisSteph | vision:masks:MinimumEigenvalueShiTomasi | vision:masks:LocalIntensityComparisonRosenDr
      mask TypeOptions thrAngle: 22.5 | 45.0 | 67.5 | 90.0 | 112.5 | 135.0 | 157.5
      mask TypeOptions output: vision:masks:CornerLocation | vision:masks:CornerLocationAndMetricMatrix | vision:masks:MetricMatrix | vision:masks:Obsolete9b
      mask TypeOptions outputInUse: vision:masks:CornerLocation | vision:masks:CornerLocationAndMetricMatrix | vision:masks:MetricMatrix
      mask TypeOptions outputMode: Same as accumulator | Same as input | Binary point scaling | Slope and bias scaling
      mask TypeOptions accumMode: Same as input | Binary point scaling | Slope and bias scaling
      mask TypeOptions prodOutputMode: Same as input | Binary point scaling | Slope and bias scaling
      mask TypeOptions memoryMode: Same as input | Binary point scaling | Slope and bias scaling
      mask TypeOptions firstCoeffMode: Same word length as input | Specify word length | Binary point scaling | Slope and bias scaling
      mask TypeOptions roundingMode: Ceiling | Convergent | Floor | Nearest | Round | Simplest | Zero
      mask Display: disp('Corner Metric');
  Find Local Maxima : visionstatistics/Find Local Maxima  num_peaks=maxNum  nhood_size=neighborSize  src_thresh=Obsolete9b  src_thresh_inuse=Specify via dialog  threshold=thrMetric  inputIsHough=off  dt_peak=uint32  isOutVarDim=on  dt_count=uint32
      settings: SourceProductName=Computer Vision System Toolbox  SourceProductBaseCode=VP
  Location : Outport
  wires:
  I/1 -> Corner Metric/1
  Corner Metric/1 -> Find Local Maxima/1
  Find Local Maxima/1 -> Location/1

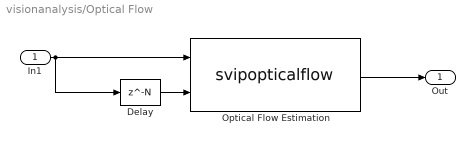
== system visionanalysis/Optical Flow ==
  In1 : Inport
  Delay : Delay  DelayLength=N
  Optical Flow Estimation : S-Function  DialogController=vipDDGCreate  FunctionName=svipopticalflow  Parameters=method,gradMethod,outVelForm,lambda,stop_criteria,maxAllowAbsDiff,maxIter,numInports,sigmaS,sigmaW,eigTh,discardNormalFlow,dtInfo.firstCoeffMode, dtInfo.firstCoeffWordLength,dtInfo.firstCoeffFracLength,dtInfo.prodOutputMode,dtInfo.prodOutputWordLength,dtInfo.prodOutputFracLength,dtInfo.accumMode,dtInfo.accumWordLength,dtInfo.accumFracLength,dtInfo.memoryMode,dtInfo.memoryWordLength,dtInfo.memoryFracLength,dtInfo.outputMode,dtInfo.outputWordLength,dtInfo.outputFracLength,dtInfo.roundingMode,dtInfo.overflowMode  SFunctionDeploymentMode=off  EnableBusSupport=off  mask(Optical Flow Estimation){method=Horn-Schunck, gradMethod=Difference filter [-1 1], which2img=Current frame and N-th frame back, N=N, outVelForm=Magnitude-squared, lambda=lambda, stop_criteria=When maximum number of iterations is reached, maxAllowAbsDiff=maxAllowAbsDiff, maxIter=maxIter, numInports=numInports, sigmaS=sigmaS, sigmaW=sigmaW, eigTh=eigTh, discardNormalFlow=off, outputCurrentImage=off, firstCoeffMode=Same word length as first input, firstCoeffWordLength=firstCoeffWordLength, firstCoeffFracLength=firstCoeffFracLength, prodOutputMode=Binary point scaling, prodOutputWordLength=prodOutputWordLength, prodOutputFracLength=prodOutputFracLength, accumMode=Same as product output, accumWordLength=accumWordLength, accumFracLength=accumFracLength, memoryMode=Same as accumulator, memoryWordLength=memoryWordLength, memoryFracLength=memoryFracLength, outputMode=Binary point scaling, outputWordLength=outputWordLength, outputFracLength=outputFracLength, roundingMode=Nearest, overflowMode=on, LockScale=off}
      mask prompts: gradMethod "Gradient method:"; which2img "Compute optical flow between:"; outVelForm "Velocity output:"; lambda "Smoothness factor:"; stop_criteria "Stop iterative solution:"; maxAllowAbsDiff "Velocity difference threshold:"; maxIter "Maximum number of iterations:"; numInports "Number of input frames to buffer:"; sigmaS "Standard deviation for image smoothing filter:"; sigmaW "Standard deviation for gradient smoothing filter:"; eigTh "Threshold for noise reduction:"; discardNormalFlow "Discard normal flow estimates when constraint equation is ill-conditioned"; outputCurrentImage "Output image corresponding to motion vectors (accounts for block delay)"; firstCoeffMode "Eigen threshold attributes:"; firstCoeffWordLength "Eigen threshold word length:"; firstCoeffFracLength "Eigen threshold fraction length:"; prodOutputMode "Product output attributes:"; prodOutputWordLength "Product output word length:"; prodOutputFracLength "Product output fraction length:"; accumMode "Accumulator attributes:"; accumWordLength "Accumulator word length:"; accumFracLength "Accumulator fraction length:"; memoryMode "Gradient attributes:"; memoryWordLength "Gradient word length:"; memoryFracLength "Gradient fraction length:"; outputMode "Fixed-point output attributes:"; outputWordLength "Output word length:"; outputFracLength "Output fractional length:"; roundingMode "Round integer calculations toward:"; overflowMode "Saturate on integer overflow"; LockScale "Lock scaling"
      mask help: Estimates optical flow between two images or two video frames.
      mask init:
      | dtInfo = dspGetFixptDataTypeInfo(gcbh,63);
      mask TypeOptions method: vision:masks:HornSchunck | vision:masks:LucasKanade
      mask TypeOptions gradMethod: vision:masks:DerivativeOfGaussian | vision:masks:DifferenceFilter
      mask TypeOptions which2img: vision:masks:TwoImages | vision:masks:CurrentFrameAndNthFrameBack
      mask TypeOptions outVelForm: vision:masks:HorizontalAndVerticalComponentsI | vision:masks:Magnitudesquared
      mask TypeOptions stop_criteria: vision:masks:WhenVelocityDifferenceFallsBelow | vision:masks:WhenMaximumNumberOfIterations | vision:masks:WhicheverComesFirst
      mask TypeOptions firstCoeffMode: Same word length as first input | Specify word length | Binary point scaling | Slope and bias scaling
      mask TypeOptions prodOutputMode: Binary point scaling | Slope and bias scaling
      mask TypeOptions accumMode: Same as product output | Binary point scaling | Slope and bias scaling
      mask TypeOptions memoryMode: Same as accumulator | Same as product output | Binary point scaling | Slope and bias scaling
      mask TypeOptions outputMode: Binary point scaling | Slope and bias scaling
      mask TypeOptions roundingMode: Ceiling | Convergent | Floor | Nearest | Round | Simplest | Zero
  Out : Outport
  wires:
  Optical Flow Estimation/1 -> Out/1
  In1/1 -> Optical Flow Estimation/1, Delay/1
  Delay/1 -> Optical Flow Estimation/2
